simulink model "Proiect6_Simulink"  (R2022b)
settings: Solver=VariableStepAuto  StartTime=0.0  StopTime=20  RelTol=1e-3
undefined symbols (not defined in the file or in its folder): denC, denH, numC, numH
settings Model: Creator=maria  LastModifiedBy=maria

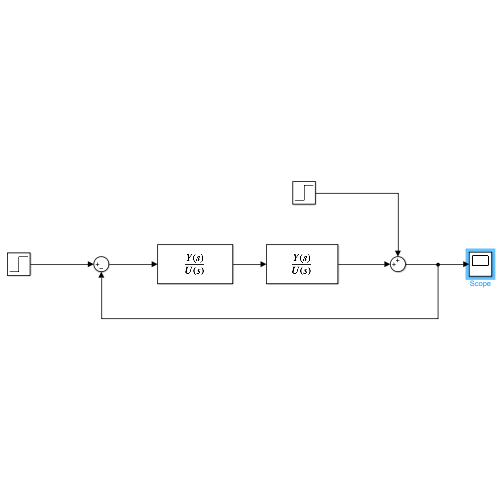
[thumbnail: Simulink's stored preview of the top-level diagram]
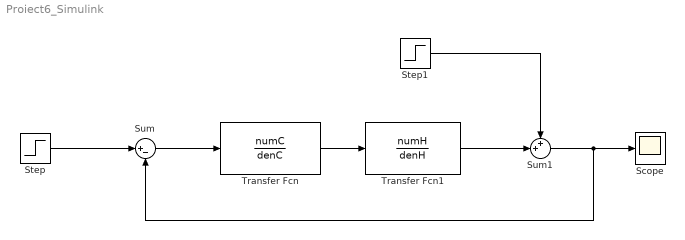
== system Proiect6_Simulink ==
  Scope : Scope
  Step : Step  Time=0  SampleTime=0
  Step1 : Step  Time=10  After=0.2  SampleTime=0
  Sum : Sum  Inputs=|+-
  Sum1 : Sum  Inputs=++|
  Transfer Fcn : TransferFcn  Numerator=numC  Denominator=denC
  Transfer Fcn1 : TransferFcn  Numerator=numH  Denominator=denH
  wires:
  Step/1 -> Sum/1
  Sum/1 -> Transfer Fcn/1
  Transfer Fcn/1 -> Transfer Fcn1/1
  Sum1/1 -> Sum/2, Scope/1
  Transfer Fcn1/1 -> Sum1/2
  Step1/1 -> Sum1/1
